simulink model "PLANET_v2"  (R2018b)
settings: Solver=FixedStepAuto  StartTime=0.0  StopTime=span-1  FixedStep=0.1  RelTol=1e-3
undefined symbols (not defined in the file): CHP_eta_el, CHP_eta_th, CHP_Pn, control, dh_demand, DH_elB_Cap, DH_elB_eff, DH_gas_B_Cap, DH_gas_B_eff, DH_HP_Cap, DH_HP_COP, DiscIntNeverNeededParam, dt, h_elD, lhd_demand, LHD_elB_Cap, LHD_elB_eff, LHD_gas_B_Cap, LHD_gas_B_eff, LHD_HP_Cap, LHD_HP_COP, Liion_cap, Liion_charge, Liion_dis, Liion_eff_ch, Liion_eff_dis, PCI, PtG_cap, PtG_eta_elcto, PtG_eta_meth, PtG_eta_th, PVPower, RES_curtailment_on_off, tt, WindPower
libraries: simulink x1
(part 1 of 5)
settings Model: Creator=Fambri  LastModifiedBy=gabriele.fambri
settings SolverCC: AlgebraicLoopSolver=LineSearch
settings DataIOCC: SaveFormat=StructureWithTime  SaveState=on  InspectSignalLogs=on
settings SFSimCC: SimUseLocalCustomCode=off
settings RTWCC: RTWUseLocalCustomCode=off
settings CodeAppCC: StateflowObjectComments=on

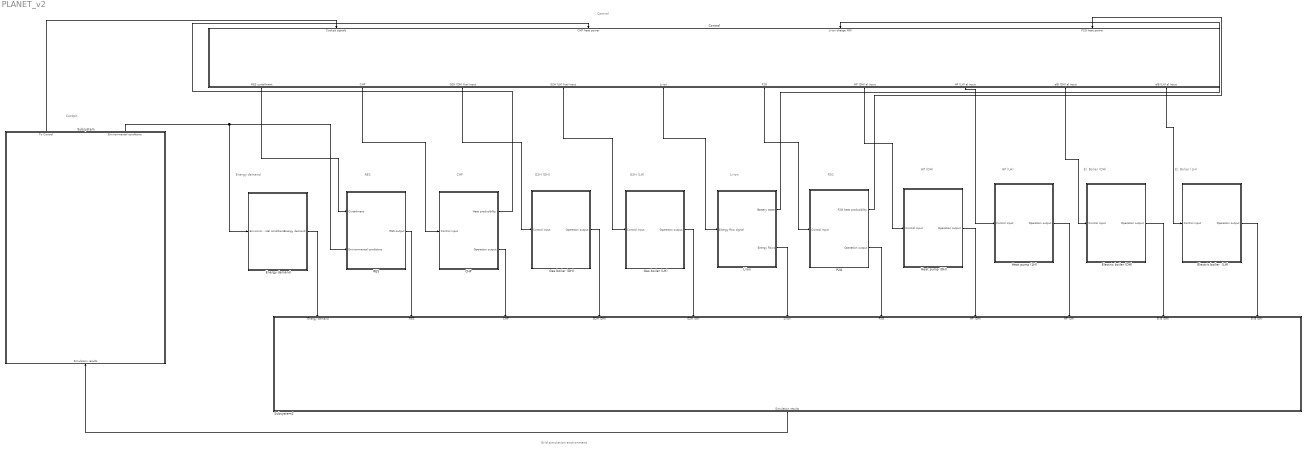
== system PLANET_v2 ==
  note: Li-ion
  note: Energy demand
  note: RES
  note: CHP
  note: P2G
  note: G2H (DH)
  note: Grid simulation environment
  note: Control
  note: HP (DH)
  note: Cockpit
  note: G2H (LH)
  note: HP (LH)
  note: El. Bolier (DH)
  note: El. Bolier (LH)
  CHP : Subsystem
  "Control " : Subsystem
  Electric boiler  (LH) : Subsystem
  Electric boiler (DH) : Subsystem
  Energy demand : Subsystem
  Gas boiler (DH) : Subsystem
  Gas boiler (LH) : Subsystem
  Heat pump (DH) : Subsystem
  Heat pump (LH) : Subsystem
  Liion : Subsystem
  P2G : Subsystem
  RES : Subsystem
  Subsystem : Subsystem
  Subsystem2 : Subsystem
  wires:
  Energy demand/1(Energy demand) -> Subsystem2/1(Energy demand)
  RES/1(RES output) -> Subsystem2/2(RES)
  Liion/2(Energy flows) -> Subsystem2/6(Li-ion)
  Gas boiler (DH)/1(Operation output) -> Subsystem2/4(G2H (DH))
  CHP/2(Operation output) -> Subsystem2/3(CHP)
  P2G/2(Operation output) -> Subsystem2/7(P2G)
  Subsystem/2(Environmental conditions) -> RES/2(Environmental conditions), Energy demand/1(Environmental conditions)
  Subsystem2/1(Simulation results) -> Subsystem/1(Simulation results)
  Subsystem/1(To Control) -> "Control "/1(Cockpit signals)
  P2G/1(P2G heat producibility) -> "Control "/4(P2G heat power)
  CHP/1(Heat producibility) -> "Control "/2(CHP heat power)
  Liion/1(Battery state) -> "Control "/3(Li-ion charge MW)
  "Control "/3("G2H (DH) fuel input ") -> Gas boiler (DH)/1(Control input)
  "Control "/1(RES curtailment) -> RES/1(Curtailment)
  "Control "/2(CHP) -> CHP/1(Control input)
  "Control "/6(P2G) -> P2G/1(Control input)
  "Control "/5(Li-ion) -> Liion/1(Energy flow signal)
  "Control "/7("HP (DH) el input ") -> Heat pump (DH)/1(Control input)
  Heat pump (DH)/1(Operation output) -> Subsystem2/8(HP (DH))
  "Control "/8("HP (LH) el input ") -> Heat pump (LH)/1(Control input)
  "Control "/9(elB (DH) el input) -> Electric boiler (DH)/1(Control input)
  "Control "/10(elB (LH) el input) -> Electric boiler  (LH)/1(Control input)
  "Control "/4(G2H (LH) fuel input) -> Gas boiler (LH)/1(Control input)
  Gas boiler (LH)/1(Operation output) -> Subsystem2/5(G2H (LH))
  Heat pump (LH)/1(Operation output) -> Subsystem2/9(HP (LH))
  Electric boiler (DH)/1(Operation output) -> Subsystem2/10(El B (DH))
  Electric boiler  (LH)/1(Operation output) -> Subsystem2/11(El B (LH))

== system PLANET_v2/CHP ==
  note: CHP fuel
  Control input : Inport
  Bus Creator : BusCreator  Inputs=3
  Bus Selector : BusSelector  OutputSignals=CHP fuel,CHP heat curtailment
  "CHP " : Subsystem  mask{PCI=PCI, eff_el=CHP_eta_el, Paus=0, eff_th=CHP_eta_th, Pn=CHP_Pn}
      mask prompts: PCI "PCI MWh/kg"; eff_el "Electric efficiency %"; Paus "Internal comsumption"; eff_th "Thermal efficiency %"; Pn "Nominal power MW"
  Sum : Sum  Inputs=|+-
  Heat producibility : Outport
  Operation output : Outport  Port=2
  wires:
  Bus Creator/1 -> Operation output/1
  "CHP "/3(Heat production) -> Heat producibility/1, Sum/1
  Sum/1 -> Bus Creator/3  "CHP heat power"
  Bus Selector/2 -> Sum/2  "<CHP heat curtailment>"
  "CHP "/1(Fuel consumption) -> Bus Creator/1
  Bus Selector/1 -> "CHP "/1(Fuel mass signal)  "<CHP fuel>"
  "CHP "/2(El production) -> Bus Creator/2  "CHP el power"
  Control input/1 -> Bus Selector/1

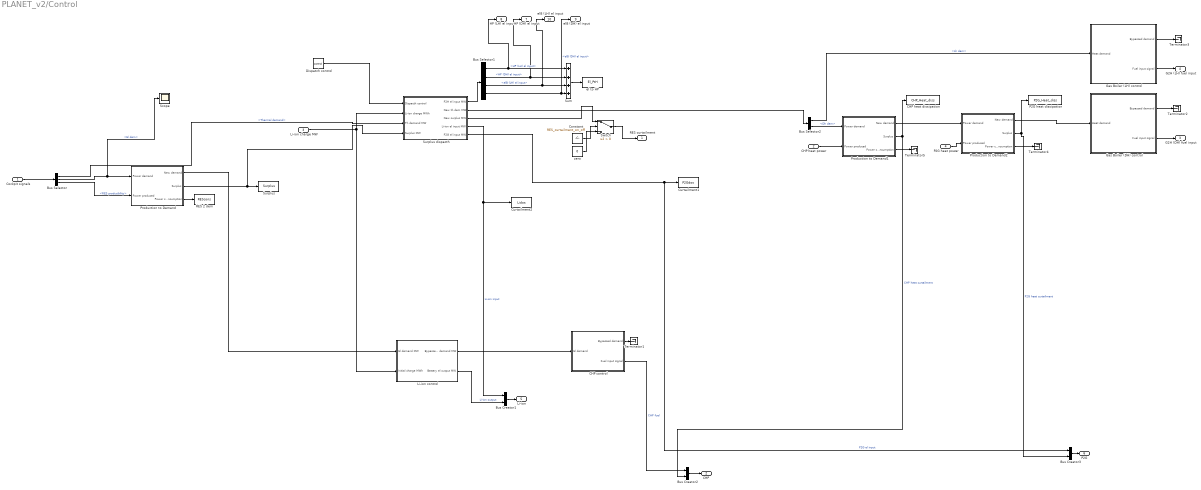
== system PLANET_v2/Control  ==
  Cockpit signals : Inport
  CHP heat power : Inport  Port=2
  Li-ion charge MW : Inport  Port=3
  P2G heat power : Inport  Port=4
  Bus Creator1 : BusCreator  Inputs=2
  Bus Creator2 : BusCreator  Inputs=2
  Bus Creator3 : BusCreator  Inputs=2
  Bus Selector : BusSelector  OutputSignals=Energy demand.Thermal demand,Energy demand.El dem,RES.RES producibility
  Bus Selector1 : BusSelector  OutputSignals=HP (LH) el input,HP (DH) el input,elB (LH) el input,elB (DH) el input
  Bus Selector2 : BusSelector  OutputSignals=Lh dem,Dh dem
  CHP control : Subsystem  mask{PCI=PCI, eff_el=CHP_eta_el, Paus=0, eff_th=CHP_eta_th, Pn=CHP_Pn}
      mask prompts: PCI "PCI MWh/kg"; eff_el "Electric efficiency %"; Paus "Internal comsumption"; eff_th "Thermal efficiency %"; Pn "Nominal power MW"
  CHP heat dissipation : ToWorkspace  VariableName=CHP_Heat_diss  SampleTime=1
  Constant : Constant  Value=RES_curtailment_on_off
  Curtailment1 : ToWorkspace  VariableName=P2Gdos  SampleTime=1
  Curtailment2 : ToWorkspace  VariableName=Lidos  SampleTime=1
  Dispatch control : Constant  Value=control
  Gas Boiler (DH) control : Subsystem  mask{PCI=PCI, eff=DH_gas_B_eff, Pn=DH_gas_B_Cap}
      mask prompts: PCI "PCI MWh/kg"; eff "Thermal efficiency %"; Pn "Nominal Power MW"
  Gas Boiler (LH) control : Subsystem  mask{PCI=PCI, eff=LHD_gas_B_eff, Pn=LHD_gas_B_Cap}
      mask prompts: PCI "PCI MWh/kg"; eff "Thermal efficiency %"; Pn "Nominal Power MW"
  Li-ion control : Subsystem  mask{eff_charge=Liion_eff_ch, eff_discharge=Liion_eff_dis, SoC_MAX=100, SoC_MIN=0, Capacity=Liion_cap, Initial_SoC=50, Max_charge=Liion_charge, Max_discharge=Liion_dis}
      mask prompts: eff_charge "charging efficiency [%]"; eff_discharge "discharging efficiency [%]"; SoC_MAX "Maximum state of charge [%]"; SoC_MIN "Minimum state of charge [%]"; Capacity "Capacity [MWh]"; Initial_SoC "Initial State of charge [%]"; Max_charge "Max charge [MW]"; Max_discharge "Max discharge [MW]"
  P2G heat dissipation : ToWorkspace  VariableName=P2G_Heat_diss  SampleTime=1
  Production to Demand : Subsystem
  Production to Demand1 : Subsystem
  Production to Demand2 : Subsystem
  RES 2 dem : ToWorkspace  VariableName=REScons  SampleTime=1
  Scope : Scope
  Sum : Sum  Inputs=++++
  Surplus : ToWorkspace  VariableName=Surplus  SampleTime=1
  Surplus dispacth : Subsystem
  Switch : Switch  Criteria=u2 > Threshold
  Terminator{1..5} (5 alike) : Terminator
  el to HP : ToWorkspace  VariableName=El_PtH  SampleTime=1
  zero : Constant  Value=0
  RES curtailment : Outport
  CHP : Outport  Port=2
  "G2H (DH) fuel input " : Outport  Port=3
  G2H (LH) fuel input : Outport  Port=4
  Li-ion : Outport  Port=5
  P2G : Outport  Port=6
  "HP (DH) el input " : Outport  Port=7
  "HP (LH) el input " : Outport  Port=8
  elB (DH) el input : Outport  Port=9
  elB (LH) el input : Outport  Port=10
  wires:
  Production to Demand/1(New demand) -> Li-ion control/1(El demand MW)
  Production to Demand/2(Surplus) -> Surplus dispacth/4(Surplus MW), Surplus/1
  Li-ion control/1(Bypassed demand MW) -> CHP control/1(El demand)
  Gas Boiler (DH) control/2(Fuel input signal) -> "G2H (DH) fuel input "/1
  Production to Demand1/2(Surplus) -> Bus Creator2/2, CHP heat dissipation/1  "CHP heat curtailment"
  Production to Demand2/1(New demand) -> Gas Boiler (DH) control/1(Heat demand)
  CHP control/2(Fuel input signal) -> Bus Creator2/1  "CHP fuel"
  Production to Demand2/2(Surplus) -> Bus Creator3/2, P2G heat dissipation/1  "P2G heat curtailment"
  P2G heat power/1 -> Production to Demand2/2(Power produced)
  Cockpit signals/1 -> Bus Selector/1
  Bus Creator2/1 -> CHP/1
  CHP heat power/1 -> Production to Demand1/2(Power produced)
  Bus Selector/3 -> Production to Demand/2(Power produced)  "<RES producibility>"
  Bus Creator1/1 -> Li-ion/1
  Li-ion control/2(Battery el output MW) -> Bus Creator1/2  "Li-ion output"
  Surplus dispacth/3(New surplus MW) -> Switch/1
  Li-ion charge MW/1 -> Li-ion control/2(Initial charge MWh), Surplus dispacth/2(Li-ion charge MWh)
  Surplus dispacth/1(P2H el input MW) -> Bus Selector1/1
  Surplus dispacth/4(Li-ion el input MW) -> Bus Creator1/1, Curtailment2/1  "Li-ion input"
  Surplus dispacth/5(P2G el input MW) -> Bus Creator3/1, Curtailment1/1  "P2G el input"
  Dispatch control/1 -> Surplus dispacth/1(Dispacth control)
  Production to Demand/3(Power consumption) -> RES 2 dem/1
  Bus Creator3/1 -> P2G/1
  Production to Demand1/1(New demand) -> Production to Demand2/1(Power demand)
  Bus Selector/2 -> Scope/1, Production to Demand/1(Power demand)  "<El dem>"
  Bus Selector/1 -> Surplus dispacth/3(Th demand MW)  "<Thermal demand>"
  Bus Selector1/2 -> Sum/2, "HP (DH) el input "/1  "<HP (DH) el input>"
  Bus Selector1/3 -> Sum/3, elB (LH) el input/1  "<elB (LH) el input>"
  Bus Selector1/4 -> elB (DH) el input/1, Sum/4  "<elB (DH) el input>"
  Sum/1 -> el to HP/1
  Surplus dispacth/2(New th dem MW) -> Bus Selector2/1
  Bus Selector2/2 -> Production to Demand1/1(Power demand)  "<Dh dem>"
  Bus Selector2/1 -> Gas Boiler (LH) control/1(Heat demand)  "<Lh dem>"
  Gas Boiler (LH) control/2(Fuel input signal) -> G2H (LH) fuel input/1
  Bus Selector1/1 -> "HP (LH) el input "/1, Sum/1  "<HP (LH) el input>"
  CHP control/1(Bypassed demand) -> Terminator1/1
  Gas Boiler (DH) control/1(Bypassed demand) -> Terminator2/1
  Gas Boiler (LH) control/1(Bypassed demand) -> Terminator3/1
  Production to Demand2/3(Power consumption) -> Terminator4/1
  Production to Demand1/3(Power consumption) -> Terminator5/1
  Constant/1 -> Switch/2
  zero/1 -> Switch/3
  Switch/1 -> RES curtailment/1

== system PLANET_v2/Electric boiler  (LH) ==
  Control input : Inport
  Bus Creator : BusCreator  Inputs=2
  Heat production : ToWorkspace  VariableName=h_P2H_elB_LH  SampleTime=1
  P2H : Subsystem  mask{COP=LHD_elB_eff, Cap=LHD_elB_Cap}
      mask prompts: COP "Efficiency/COP"; Cap "Capacity"
  Operation output : Outport
  wires:
  Control input/1 -> P2H/1(El input)
  P2H/2(heat) -> Bus Creator/2, Heat production/1  "elB (LH) heat production"
  P2H/1(El consumption) -> Bus Creator/1  "elB (LH) el input"
  Bus Creator/1 -> Operation output/1  "elB (LH) data"

== system PLANET_v2/Electric boiler (DH) ==
  Control input : Inport
  Bus Creator : BusCreator  Inputs=2
  Heat production : ToWorkspace  VariableName=h_P2H_elB_DH  SampleTime=1
  P2H : Subsystem  mask{COP=DH_elB_eff, Cap=DH_elB_Cap}
      mask prompts: COP "Efficiency/COP"; Cap "Capacity"
  Operation output : Outport
  wires:
  Control input/1 -> P2H/1(El input)
  P2H/2(heat) -> Heat production/1, Bus Creator/2  "elB (DH) heat production"
  P2H/1(El consumption) -> Bus Creator/1  "elB (DH) el input"
  Bus Creator/1 -> Operation output/1  "elB (DH) data"

== system PLANET_v2/Energy demand ==
  Environmental conditions : Inport
  Bus Creator : BusCreator  Inputs=2
  Bus Creator1 : BusCreator  Inputs=2
  Bus Selector : BusSelector  OutputSignals=El dem,DH standar profile,LH standard profile
  DH demand : Subsystem
  El demand : Subsystem
  LH demand : Subsystem
  Energy demand : Outport
  wires:
  Environmental conditions/1 -> Bus Selector/1
  DH demand/1(DH demand) -> Bus Creator1/1  "Dh dem"
  Bus Creator/1 -> Energy demand/1
  Bus Selector/1 -> El demand/1(In1)  "<El dem>"
  El demand/1(El demand) -> Bus Creator/1  "El dem"
  LH demand/1(DH demand) -> Bus Creator1/2  "Lh dem"
  Bus Creator1/1 -> Bus Creator/2  "Thermal demand"
  Bus Selector/2 -> DH demand/1(In1)  "<DH standar profile>"
  Bus Selector/3 -> LH demand/1(In1)  "<LH standard profile>"

== system PLANET_v2/Gas boiler (DH) ==
  Control input : Inport
  Bus Creator : BusCreator  Inputs=2
  DH Gas Boiler block : Subsystem  mask{PCI=PCI, eff=DH_gas_B_eff, Pn=DH_gas_B_Cap}
      mask prompts: PCI "PCI MWh/kg"; eff "Thermal efficiency %"; Pn "Nominal Power MW"
  Operation output : Outport
  wires:
  Bus Creator/1 -> Operation output/1  "G2H (DH) data"
  DH Gas Boiler block/2(Thermal power) -> Bus Creator/2  "DG2H heat"
  DH Gas Boiler block/1("Fuel mass ") -> Bus Creator/1  "DG2H fuel"
  Control input/1 -> DH Gas Boiler block/1(Fuel mass signal)

== system PLANET_v2/Gas boiler (LH) ==
  Control input : Inport
  Bus Creator : BusCreator  Inputs=2
  LH Gas Boiler block : Subsystem  mask{PCI=PCI, eff=LHD_gas_B_eff, Pn=LHD_gas_B_Cap}
      mask prompts: PCI "PCI MWh/kg"; eff "Thermal efficiency %"; Pn "Nominal Power MW"
  Operation output : Outport
  wires:
  Bus Creator/1 -> Operation output/1  "G2H (LH) data"
  LH Gas Boiler block/2(Thermal power) -> Bus Creator/2  "LG2H heat"
  LH Gas Boiler block/1("Fuel mass ") -> Bus Creator/1  "LG2H fuel"
  Control input/1 -> LH Gas Boiler block/1(Fuel mass signal)

== system PLANET_v2/Heat pump (DH) ==
  Control input : Inport
  Bus Creator : BusCreator  Inputs=2
  Heat production : ToWorkspace  VariableName=h_P2H_HP_DH  SampleTime=1
  P2H : Subsystem  mask{COP=DH_HP_COP, Cap=DH_HP_Cap}
      mask prompts: COP "Efficiency/COP"; Cap "Capacity"
  Operation output : Outport
  wires:
  Control input/1 -> P2H/1(El input)
  P2H/2(heat) -> Heat production/1, Bus Creator/2  "DHP heat production"
  P2H/1(El consumption) -> Bus Creator/1  "DHP el input"
  Bus Creator/1 -> Operation output/1  "HP (DH) data"

== system PLANET_v2/Heat pump (LH) ==
  Control input : Inport
  Bus Creator : BusCreator  Inputs=2
  Heat production : ToWorkspace  VariableName=h_P2H_HP_LH  SampleTime=1
  P2H : Subsystem  mask{COP=LHD_HP_COP, Cap=LHD_HP_Cap}
      mask prompts: COP "Efficiency/COP"; Cap "Capacity"
  Operation output : Outport
  wires:
  Control input/1 -> P2H/1(El input)
  P2H/2(heat) -> Heat production/1, Bus Creator/2  "LHP heat production"
  P2H/1(El consumption) -> Bus Creator/1  "LHP el input"
  Bus Creator/1 -> Operation output/1  "HP (LH) data"

== system PLANET_v2/Liion ==
  note: Li-ion input
  Energy flow signal : Inport
  Bus Creator : BusCreator  Inputs=2
  Bus Selector : BusSelector  OutputSignals=Li-ion input,Li-ion output
  "Li-ion " : Subsystem  mask{eff_charge=Liion_eff_ch, eff_discharge=Liion_eff_dis, SoC_MAX=100, SoC_MIN=0, Capacity=Liion_cap, Initial_SoC=50, Max_charge=Liion_charge, Max_discharge=Liion_dis, Parameter11=<empty>}
      mask prompts: eff_charge "charging efficiency [%]"; eff_discharge "discharging efficiency [%]"; SoC_MAX "Maximum state of charge [%]"; SoC_MIN "Minimum state of charge [%]"; Capacity "Capacity [MWh]"; Initial_SoC "Initial State of charge [%]"; Max_charge "Max charge [MW]"; Max_discharge "Max discharge [MW]"
      mask TypeOptions Parameter11: <empty>
  Battery state : Outport
  Energy flows : Outport  Port=2
  wires:
  Energy flow signal/1 -> Bus Selector/1
  "Li-ion "/1(Initial Charge) -> Battery state/1
  Bus Creator/1 -> Energy flows/1
  "Li-ion "/2(El consumption) -> Bus Creator/1
  "Li-ion "/3(El production) -> Bus Creator/2  "Li-ion output"
  Bus Selector/1 -> "Li-ion "/1(El input)  "<Li-ion input>"
  Bus Selector/2 -> "Li-ion "/2(El output)  "<Li-ion output>"

== system PLANET_v2/P2G ==
  Control input : Inport
  Bus Creator : BusCreator  Inputs=3
  Bus Selector : BusSelector  OutputSignals=P2G el input,P2G heat curtailment
  P2G : Subsystem  mask{PtG_capacity=PtG_cap, eff_electrolyser=PtG_eta_elcto, eff_methanizer=PtG_eta_meth, eff_thermal=PtG_eta_th, PCI=PCI}
      mask prompts: PtG_capacity "PtG capacity"; eff_electrolyser "Electrolyser efficiency"; eff_methanizer "Methanizer efficiency"; eff_thermal "Thermal efficiency"; PCI "PCI Mehtane MWh/kg"
  Sum2 : Sum  Inputs=|+-
  P2G heat producibility : Outport
  Operation output : Outport  Port=2
  wires:
  Bus Creator/1 -> Operation output/1
  P2G/2(El consumption) -> Bus Creator/2  "P2G el imput"
  Sum2/1 -> Bus Creator/3  "P2G heat production"
  Bus Selector/2 -> Sum2/2  "<P2G heat curtailment>"
  P2G/1(Gas productioon) -> Bus Creator/1  "P2G gas production"
  P2G/3(Heat production) -> P2G heat producibility/1, Sum2/1
  Bus Selector/1 -> P2G/1(El input)  "<P2G el input>"
  Control input/1 -> Bus Selector/1

== system PLANET_v2/RES ==
  Curtailment : Inport
  Environmental conditions : Inport  Port=2
  Bus Creator : BusCreator  Inputs=3
  Bus Selector : BusSelector  OutputSignals=Wind,PV,Hydro
  Subsystem : Subsystem
  Sum1 : Sum  Inputs=-+|
  Sum3 : Sum  Inputs=+++
  RES output : Outport
  wires:
  Sum3/1 -> Sum1/2, Bus Creator/3  "RES producibility"
  Subsystem/2(RES2) -> Sum3/2
  Subsystem/1(RES1) -> Sum3/1
  Subsystem/3(RES3) -> Sum3/3
  Bus Selector/1 -> Subsystem/1(Wind)  "<Wind>"
  Bus Selector/2 -> Subsystem/2(PV)  "<PV>"
  Sum1/1 -> Bus Creator/2  "RES production"
  Curtailment/1 -> Bus Creator/1, Sum1/1  "Curtailment"
  Bus Creator/1 -> RES output/1
  Environmental conditions/1 -> Bus Selector/1
  Bus Selector/3 -> Subsystem/3(Hydro)  "<Hydro>"

== system PLANET_v2/Subsystem ==
  Simulation results : Inport
  Environment : Subsystem
  To Matlab : Subsystem
  To Control : Outport
  Environmental conditions : Outport  Port=2
  wires:
  Simulation results/1 -> To Matlab/1(Simulation results), To Control/1
  Environment/1(Environmental conditions) -> Environmental conditions/1

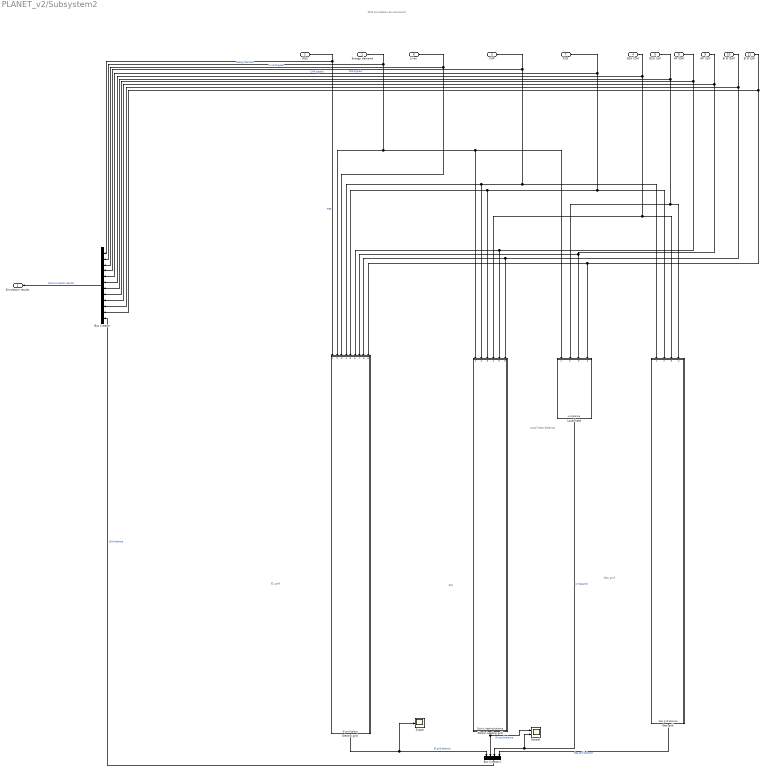
== system PLANET_v2/Subsystem2 ==
  note: EL grid
  note: DH
  note: Local heat balance
  note: Gas grid
  note: Grid simulation environment
  Energy demand : Inport
  RES : Inport  Port=2
  CHP : Inport  Port=3
  G2H (DH) : Inport  Port=4
  G2H (LH) : Inport  Port=5
  Li-ion : Inport  Port=6
  P2G : Inport  Port=7
  HP (DH) : Inport  Port=8
  HP (LH) : Inport  Port=9
  El B (DH) : Inport  Port=10
  El B (LH) : Inport  Port=11
  Bus Creator : BusCreator  Inputs=12
  Bus Creator1 : BusCreator  Inputs=4
  Distric heating grid : Subsystem
  Electric grid : Subsystem
  Gas grid : Subsystem
  Local heat : Subsystem
  Scope : Scope
  Scope1 : Scope  NumInputPorts=2
  Simulation results : Outport
  wires:
  G2H (DH)/1 -> Gas grid/3(Gas boiler (DH)), Distric heating grid/4(Gas boiler (DH)), Bus Creator/6
  Bus Creator/1 -> Simulation results/1  "Grid simulation results"
  Electric grid/1(El grid balace) -> Scope/1, Bus Creator1/1  "El grid balance"
  Energy demand/1 -> Distric heating grid/1(Demand consumption), Local heat/1(LH dem), Electric grid/2(Demand consumption), Bus Creator/2  "Energy demand"
  CHP/1 -> Gas grid/1(CHP consumption), Electric grid/4(CHP production), Distric heating grid/2(CHP production), Bus Creator/4  "CHP signals"
  Bus Creator1/1 -> Bus Creator/12  "Grid balance"
  P2G/1 -> Electric grid/5(P2G consumption), Distric heating grid/3(P2G production), Gas grid/2(P2G production), Bus Creator/5  "P2G signals"
  Distric heating grid/1(Distric heating balance) -> Scope1/1, Bus Creator1/2  "DH grid balance"
  Gas grid/1(Gas grid balance) -> Bus Creator1/4  "Gas grid balance"
  Li-ion/1 -> Electric grid/3(Li-ion), Bus Creator/3  "Li-ion signals"
  HP (DH)/1 -> Electric grid/6(HP (DH) el), Distric heating grid/5(HP (DH)), Bus Creator/8
  RES/1 -> Bus Creator/1, Electric grid/1(RES)  "RES"
  Local heat/1(LH balance) -> Scope1/2, Bus Creator1/3  "LH balance"
  G2H (LH)/1 -> Local heat/2(Gas boiler (LH)), Gas grid/4(Gas boiler (LH)), Bus Creator/7
  HP (LH)/1 -> Local heat/3(HP (LH)), Electric grid/7(HP (LH) el), Bus Creator/9
  El B (DH)/1 -> Electric grid/8(El B (DH) el), Distric heating grid/6(El B (DH)), Bus Creator/10
  El B (LH)/1 -> Electric grid/9(El B (LH) el), Local heat/4(El B (LH)), Bus Creator/11

== system PLANET_v2/CHP/CHP  ==
  Fuel mass signal : Inport
  CHP : Subsystem
  Fuel consumption : Outport
  El production : Outport  Port=2
  Heat production : Outport  Port=3
  wires:
  CHP/1(Electric power) -> El production/1
  Fuel mass signal/1 -> Fuel consumption/1, CHP/1(Fuel mass flow rate)
  CHP/2(Thermal power) -> Heat production/1

== system PLANET_v2/Control /CHP control ==
  El demand : Inport
  Divide1 : Product  Inputs=*/
  Divide2 : Product  Inputs=**
  Electric efficiency : Constant  Value=eff_el/100
  Internal comsumption : Constant  Value=Paus
  Nominal CHP power : Constant  Value=Pn
  PCI MJ/kg1 : Constant  Value=PCI
  Saturation : Saturate  UpperLimit=Pn/PCI/(eff_el/100)  LowerLimit=0
  Saturation1 : Saturate  UpperLimit=inf  LowerLimit=0
  Sum1 : Sum  Inputs=++|
  Sum2 : Sum  Inputs=-+|
  Bypassed demand : Outport
  Fuel input signal : Outport  Port=2
  wires:
  Sum1/1 -> Divide1/1
  Internal comsumption/1 -> Sum1/1
  Electric efficiency/1 -> Divide2/2
  Sum2/1 -> Saturation1/1
  Saturation/1 -> Fuel input signal/1
  El demand/1 -> Sum2/2, Sum1/2
  Saturation1/1 -> Bypassed demand/1
  PCI MJ/kg1/1 -> Divide2/1
  Divide2/1 -> Divide1/2
  Nominal CHP power/1 -> Sum2/1
  Divide1/1 -> Saturation/1

== system PLANET_v2/Control /Gas Boiler (DH) control ==
  Heat demand : Inport
  Divide1 : Product  Inputs=*/
  Divide2 : Product  Inputs=**
  Nominal Gas boiler power : Constant  Value=Pn
  PCI MJ/kg1 : Constant  Value=PCI
  Saturation : Saturate  UpperLimit=Pn/PCI/(eff/100)  LowerLimit=0
  Saturation1 : Saturate  UpperLimit=inf  LowerLimit=0
  Sum4 : Sum  Inputs=-+|
  thermal efficiency : Constant  Value=eff/100
  Bypassed demand : Outport
  Fuel input signal : Outport  Port=2
  wires:
  Divide1/1 -> Saturation/1
  Divide2/1 -> Divide1/2
  Saturation/1 -> Fuel input signal/1
  Sum4/1 -> Saturation1/1
  PCI MJ/kg1/1 -> Divide2/1
  Saturation1/1 -> Bypassed demand/1
  thermal efficiency/1 -> Divide2/2
  Nominal Gas boiler power/1 -> Sum4/1
  Heat demand/1 -> Divide1/1, Sum4/2

== system PLANET_v2/Control /Gas Boiler (LH) control ==
  Heat demand : Inport
  Divide1 : Product  Inputs=*/
  Divide2 : Product  Inputs=**
  Nominal Gas boiler power : Constant  Value=Pn
  PCI MJ/kg1 : Constant  Value=PCI
  Saturation : Saturate  UpperLimit=Pn/PCI/(eff/100)  LowerLimit=0
  Saturation1 : Saturate  UpperLimit=inf  LowerLimit=0
  Scope : Scope  NumInputPorts=2
  Sum4 : Sum  Inputs=-+|
  thermal efficiency : Constant  Value=eff/100
  Bypassed demand : Outport
  Fuel input signal : Outport  Port=2
  wires:
  Divide1/1 -> Scope/1, Saturation/1
  Divide2/1 -> Divide1/2
  Saturation/1 -> Scope/2, Fuel input signal/1
  Sum4/1 -> Saturation1/1
  PCI MJ/kg1/1 -> Divide2/1
  Saturation1/1 -> Bypassed demand/1
  thermal efficiency/1 -> Divide2/2
  Nominal Gas boiler power/1 -> Sum4/1
  Heat demand/1 -> Divide1/1, Sum4/2

== system PLANET_v2/Control /Li-ion control ==
  El demand MW : Inport
  Initial charge MWh : Inport  Port=2
  Available Energy MWh : Subsystem
  Bypassed dem : Merge  Inputs=4
  Disch eff : Gain  Gain=eff_discharge/100
  Energy to Power : Subsystem
  From battery : Merge  Inputs=4
  If Action Subsystem3 : Subsystem  TreatAsAtomicUnit=on
  If Action Subsystem5 : Subsystem  TreatAsAtomicUnit=on
  If Action Subsystem6 : Subsystem  TreatAsAtomicUnit=on
  If Action Subsystem7 : Subsystem  TreatAsAtomicUnit=on
  Max discharge rate MW : Subsystem
  if demand : If  NumInputs=3  IfExpression=u1 == 0  ElseIfExpressions=(u1 <= u2) & (u1<=u3), u2<=u3
  Bypassed demand MW : Outport
  Battery el output MW : Outport  Port=2
  wires:
  if demand/4 -> If Action Subsystem7/Action
  Bypassed dem/1 -> Bypassed demand MW/1  "Unsatisfied demandt"
  If Action Subsystem5/1(From battery) -> From battery/2
  Available Energy MWh/1(Charge available) -> Energy to Power/1(Energy)
  if demand/1 -> If Action Subsystem3/Action
  If Action Subsystem7/2(Bypassed demand) -> Bypassed dem/4
  Max discharge rate MW/1(Max battery discharge) -> If Action Subsystem6/1(Max discharge), if demand/2
  If Action Subsystem5/2(Bypassed demand) -> Bypassed dem/2
  if demand/2 -> If Action Subsystem5/Action
  From battery/1 -> Battery el output MW/1  "Energy coming from the battery"
  If Action Subsystem6/2(Bypassed demand) -> Bypassed dem/3
  If Action Subsystem7/1(From battery) -> From battery/4
  if demand/3 -> If Action Subsystem6/Action
  If Action Subsystem3/2("Bypassed demand ") -> Bypassed dem/1
  If Action Subsystem6/1(From battery) -> From battery/3
  If Action Subsystem3/1(From battery) -> From battery/1
  El demand MW/1 -> If Action Subsystem7/2(Demnad), If Action Subsystem6/2(Demand), if demand/1, If Action Subsystem5/1(Demand)
  Initial charge MWh/1 -> Available Energy MWh/1(In1)
  Energy to Power/1(Power) -> Disch eff/1
  Disch eff/1 -> If Action Subsystem7/1(Available battery), if demand/3

== system PLANET_v2/Control /Production to Demand ==
  Power demand : Inport
  Power produced : Inport  Port=2
  If : If  NumInputs=2  IfExpression=u1 >= u2
  If Action Subsystem : Subsystem  TreatAsAtomicUnit=on
  If Action Subsystem1 : Subsystem  TreatAsAtomicUnit=on
  Merge : Merge
  Merge1 : Merge
  Sum : Sum  Inputs=|+-
  New demand : Outport
  Surplus : Outport  Port=2
  Power consumption : Outport  Port=3
  wires:
  Power demand/1 -> If Action Subsystem1/2(Power demand), If Action Subsystem/2(Power demand), If/2
  Power produced/1 -> Sum/1, If Action Subsystem1/1(Power produced), If Action Subsystem/1(Power produced), If/1
  If/1 -> If Action Subsystem/Action
  If/2 -> If Action Subsystem1/Action
  Merge/1 -> Sum/2, Surplus/1
  If Action Subsystem/2(Surplus) -> Merge/1
  If Action Subsystem1/1(Surplus) -> Merge/2
  If Action Subsystem/1(New demand) -> Merge1/1
  If Action Subsystem1/2(New demand) -> Merge1/2
  Merge1/1 -> New demand/1
  Sum/1 -> Power consumption/1

== system PLANET_v2/Control /Production to Demand1 ==
  Power demand : Inport
  Power produced : Inport  Port=2
  If : If  NumInputs=2  IfExpression=u1 >= u2
  If Action Subsystem : Subsystem  TreatAsAtomicUnit=on
  If Action Subsystem1 : Subsystem  TreatAsAtomicUnit=on
  Merge : Merge
  Merge1 : Merge
  Sum : Sum  Inputs=|+-
  New demand : Outport
  Surplus : Outport  Port=2
  Power consumption : Outport  Port=3
  wires:
  Power demand/1 -> If Action Subsystem1/2(Power demand), If Action Subsystem/2(Power demand), If/2
  Power produced/1 -> Sum/1, If Action Subsystem1/1(Power produced), If Action Subsystem/1(Power produced), If/1
  If/1 -> If Action Subsystem/Action
  If/2 -> If Action Subsystem1/Action
  Merge/1 -> Sum/2, Surplus/1
  If Action Subsystem/2(Surplus) -> Merge/1
  If Action Subsystem1/1(Surplus) -> Merge/2
  If Action Subsystem/1(New demand) -> Merge1/1
  If Action Subsystem1/2(New demand) -> Merge1/2
  Merge1/1 -> New demand/1
  Sum/1 -> Power consumption/1

== system PLANET_v2/Control /Production to Demand2 ==
  Power demand : Inport
  Power produced : Inport  Port=2
  If : If  NumInputs=2  IfExpression=u1 >= u2
  If Action Subsystem : Subsystem  TreatAsAtomicUnit=on
  If Action Subsystem1 : Subsystem  TreatAsAtomicUnit=on
  Merge : Merge
  Merge1 : Merge
  Sum : Sum  Inputs=|+-
  New demand : Outport
  Surplus : Outport  Port=2
  Power consumption : Outport  Port=3
  wires:
  Power demand/1 -> If Action Subsystem1/2(Power demand), If Action Subsystem/2(Power demand), If/2
  Power produced/1 -> Sum/1, If Action Subsystem1/1(Power produced), If Action Subsystem/1(Power produced), If/1
  If/1 -> If Action Subsystem/Action
  If/2 -> If Action Subsystem1/Action
  Merge/1 -> Sum/2, Surplus/1
  If Action Subsystem/2(Surplus) -> Merge/1
  If Action Subsystem1/1(Surplus) -> Merge/2
  If Action Subsystem/1(New demand) -> Merge1/1
  If Action Subsystem1/2(New demand) -> Merge1/2
  Merge1/1 -> New demand/1
  Sum/1 -> Power consumption/1

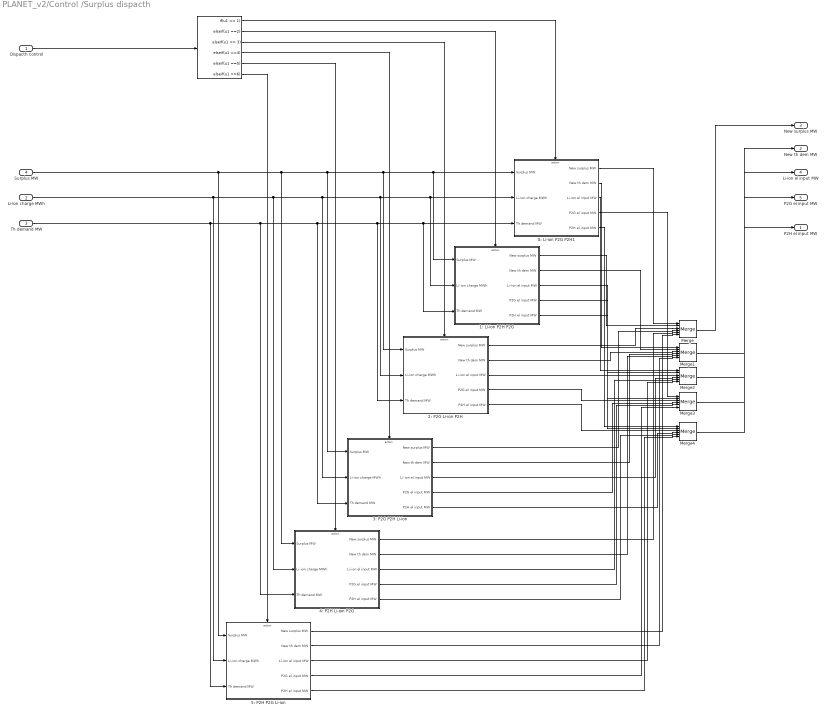
== system PLANET_v2/Control /Surplus dispacth ==
  Dispacth control : Inport
  Li-ion charge MWh : Inport  Port=2
  Th demand MW : Inport  Port=3
  Surplus MW : Inport  Port=4
  " " : If  IfExpression=u1 == 1  ElseIfExpressions=u1 ==2, u1 == 3, u1 ==4, u1 ==5, u1 ==6  ShowElse=off
  0: Li-ion P2G P2H1 : Subsystem  TreatAsAtomicUnit=on
  1: Li-ion P2H P2G : Subsystem  TreatAsAtomicUnit=on
  2: P2G Li-ion P2H : Subsystem  TreatAsAtomicUnit=on
  3: P2G P2H Li-ion : Subsystem  TreatAsAtomicUnit=on
  4: P2H Li-ion P2G : Subsystem  TreatAsAtomicUnit=on
  "5: P2H P2G Li-ion " : Subsystem  TreatAsAtomicUnit=on
  Merge{,1..4} (5 alike) : Merge  Inputs=6
  P2H el input MW : Outport
  New th dem MW : Outport  Port=2
  New surplus MW : Outport  Port=3
  Li-ion el input MW : Outport  Port=4
  P2G el input MW : Outport  Port=5
  wires:
  Merge/1 -> New surplus MW/1
  Dispacth control/1 -> " "/1
  " "/6 -> "5: P2H P2G Li-ion "/Action
  " "/5 -> 4: P2H Li-ion P2G/Action
  " "/4 -> 3: P2G P2H Li-ion/Action
  " "/3 -> 2: P2G Li-ion P2H/Action
  " "/2 -> 1: Li-ion P2H P2G/Action
  " "/1 -> 0: Li-ion P2G P2H1/Action
  Merge4/1 -> P2H el input MW/1
  Merge3/1 -> P2G el input MW/1
  Merge2/1 -> Li-ion el input MW/1
  Merge1/1 -> New th dem MW/1
  "5: P2H P2G Li-ion "/5(P2H el input MW) -> Merge4/6
  1: Li-ion P2H P2G/5(P2H el input MW) -> Merge4/2
  4: P2H Li-ion P2G/5(P2H el input MW) -> Merge4/5
  3: P2G P2H Li-ion/5(P2H el input MW) -> Merge4/4
  2: P2G Li-ion P2H/5(P2H el input MW) -> Merge4/3
  0: Li-ion P2G P2H1/5(P2H el input MW) -> Merge4/1
  "5: P2H P2G Li-ion "/4(P2G el input MW) -> Merge3/6
  4: P2H Li-ion P2G/4(P2G el input MW) -> Merge3/5
  3: P2G P2H Li-ion/4(P2G el input MW) -> Merge3/4
  2: P2G Li-ion P2H/4(P2G el input MW) -> Merge3/3
  1: Li-ion P2H P2G/4(P2G el input MW) -> Merge3/2
  0: Li-ion P2G P2H1/4(P2G el input MW) -> Merge3/1
  "5: P2H P2G Li-ion "/3(Li-ion el input MW) -> Merge2/6
  4: P2H Li-ion P2G/3(Li-ion el input MW) -> Merge2/5
  3: P2G P2H Li-ion/3(Li-ion el input MW) -> Merge2/4
  2: P2G Li-ion P2H/3(Li-ion el input MW) -> Merge2/3
  1: Li-ion P2H P2G/3(Li-ion el input MW) -> Merge2/2
  0: Li-ion P2G P2H1/3(Li-ion el input MW) -> Merge2/1
  "5: P2H P2G Li-ion "/2(New th dem MW) -> Merge1/6
  4: P2H Li-ion P2G/2(New th dem MW) -> Merge1/5
  3: P2G P2H Li-ion/2(New th dem MW) -> Merge1/4
  2: P2G Li-ion P2H/2(New th dem MW) -> Merge1/3
  1: Li-ion P2H P2G/2(New th dem MW) -> Merge1/2
  0: Li-ion P2G P2H1/2(New th dem MW) -> Merge1/1
  "5: P2H P2G Li-ion "/1(New surplus MW) -> Merge/6
  4: P2H Li-ion P2G/1(New surplus MW) -> Merge/5
  3: P2G P2H Li-ion/1(New surplus MW) -> Merge/4
  2: P2G Li-ion P2H/1(New surplus MW) -> Merge/3
  1: Li-ion P2H P2G/1(New surplus MW) -> Merge/2
  0: Li-ion P2G P2H1/1(New surplus MW) -> Merge/1
  Th demand MW/1 -> 0: Li-ion P2G P2H1/3(Th demand MW), 1: Li-ion P2H P2G/3(Th demand MW), 2: P2G Li-ion P2H/3(Th demand MW), 3: P2G P2H Li-ion/3(Th demand MW), 4: P2H Li-ion P2G/3(Th demand MW), "5: P2H P2G Li-ion "/3(Th demand MW)
  Li-ion charge MWh/1 -> 0: Li-ion P2G P2H1/2(" Li-ion charge MWh"), 1: Li-ion P2H P2G/2(" Li-ion charge MWh"), 2: P2G Li-ion P2H/2(" Li-ion charge MWh"), 3: P2G P2H Li-ion/2(" Li-ion charge MWh"), 4: P2H Li-ion P2G/2(" Li-ion charge MWh"), "5: P2H P2G Li-ion "/2(" Li-ion charge MWh")
  Surplus MW/1 -> 0: Li-ion P2G P2H1/1(Surplus MW), 1: Li-ion P2H P2G/1(Surplus MW), 2: P2G Li-ion P2H/1(Surplus MW), 3: P2G P2H Li-ion/1(Surplus MW), 4: P2H Li-ion P2G/1(Surplus MW), "5: P2H P2G Li-ion "/1(Surplus MW)

== system PLANET_v2/Electric boiler  (LH)/P2H ==
  El input : Inport
  Gain : Gain  Gain=COP
  Saturation : Saturate  UpperLimit=Cap  LowerLimit=0
  El consumption : Outport
  heat : Outport  Port=2
  wires:
  Gain/1 -> heat/1
  Saturation/1 -> Gain/1
  El input/1 -> El consumption/1, Saturation/1

== system PLANET_v2/Electric boiler (DH)/P2H ==
  El input : Inport
  Gain : Gain  Gain=COP
  Saturation : Saturate  UpperLimit=Cap  LowerLimit=0
  El consumption : Outport
  heat : Outport  Port=2
  wires:
  Gain/1 -> heat/1
  Saturation/1 -> Gain/1
  El input/1 -> El consumption/1, Saturation/1

== system PLANET_v2/Energy demand/DH demand ==
  In1 : Inport
  DH demand : Outport
  wires:
  In1/1 -> DH demand/1

== system PLANET_v2/Energy demand/El demand ==
  In1 : Inport
  El demand : Outport
  wires:
  In1/1 -> El demand/1

== system PLANET_v2/Energy demand/LH demand ==
  In1 : Inport
  DH demand : Outport
  wires:
  In1/1 -> DH demand/1

== system PLANET_v2/Gas boiler (DH)/DH Gas Boiler block ==
  Fuel mass signal : Inport
  Boiler : Subsystem
  Saturation : Saturate  UpperLimit=Pn/PCI/(eff/100)  LowerLimit=0
  "Fuel mass " : Outport
  Thermal power : Outport  Port=2
  wires:
  Boiler/1(Thermal power) -> Thermal power/1
  Fuel mass signal/1 -> Saturation/1
  Saturation/1 -> "Fuel mass "/1, Boiler/1(Fuel mass)

== system PLANET_v2/Gas boiler (LH)/LH Gas Boiler block ==
  Fuel mass signal : Inport
  Boiler : Subsystem
  Saturation : Saturate  UpperLimit=Pn/PCI/(eff/100)  LowerLimit=0
  "Fuel mass " : Outport
  Thermal power : Outport  Port=2
  wires:
  Boiler/1(Thermal power) -> Thermal power/1
  Saturation/1 -> "Fuel mass "/1, Boiler/1(Fuel mass)
  Fuel mass signal/1 -> Saturation/1

== system PLANET_v2/Heat pump (DH)/P2H ==
  El input : Inport
  Gain : Gain  Gain=COP
  Saturation : Saturate  UpperLimit=Cap  LowerLimit=0
  El consumption : Outport
  heat : Outport  Port=2
  wires:
  Gain/1 -> heat/1
  Saturation/1 -> Gain/1
  El input/1 -> El consumption/1, Saturation/1

== system PLANET_v2/Heat pump (LH)/P2H ==
  El input : Inport
  Gain : Gain  Gain=COP
  Saturation : Saturate  UpperLimit=Cap  LowerLimit=0
  El consumption : Outport
  heat : Outport  Port=2
  wires:
  Gain/1 -> heat/1
  Saturation/1 -> Gain/1
  El input/1 -> El consumption/1, Saturation/1

== system PLANET_v2/Liion/Li-ion  ==
  El input : Inport
  El output : Inport  Port=2
  1/Dis eff : Gain  Gain=100/eff_discharge
  Ch eff : Gain  Gain=eff_charge/100
  Li-ion Charge : ToWorkspace  VariableName=Liion_Charge1  SampleTime=1
  SoC Liion : ToWorkspace  VariableName=SoC_Liion1  SampleTime=1
  State of charge calulation : Subsystem
  Subsystem : Subsystem
  Initial Charge : Outport
  El consumption : Outport  Port=2
  El production : Outport  Port=3
  wires:
  El input/1 -> Ch eff/1, El consumption/1
  Subsystem/1("Initial charge ") -> Initial Charge/1
  El output/1 -> El production/1, 1/Dis eff/1
  State of charge calulation/1(State of Charege) -> SoC Liion/1
  Subsystem/2(New charge) -> State of charge calulation/1(Charge), Li-ion Charge/1
  Ch eff/1 -> Subsystem/1(El input)
  1/Dis eff/1 -> Subsystem/2(El output)

== system PLANET_v2/P2G/P2G ==
  El input : Inport
  Constant : Constant  Value=0
  Eff electrolyser : Gain  Gain=eff_electrolyser/100
  Eff methaniser : Gain  Gain=eff_methanizer/100
  Eff thermal : Gain  Gain=eff_thermal/100
  Max P2G electric input : Subsystem
  PCI : Gain  Gain=1/PCI
  Saturation Dynamic : simulink/Discontinuities/Saturation Dynamic  OutMin=0  OutMax=[]  OutDataTypeStr=Inherit: Same as second input  OutDataType=fixdt(1, 16)  OutScaling=2^-10  DoSatur=off
  Gas productioon : Outport
  El consumption : Outport  Port=2
  Heat production : Outport  Port=3
  wires:
  Max P2G electric input/1(Max P2G input) -> Saturation Dynamic/1
  Eff electrolyser/1 -> Eff methaniser/1  "H2 Power"
  Eff thermal/1 -> Heat production/1
  Eff methaniser/1 -> PCI/1  "CH4 Power"
  PCI/1 -> Gas productioon/1
  Saturation Dynamic/1 -> El consumption/1, Eff thermal/1, Eff electrolyser/1
  El input/1 -> Saturation Dynamic/2
  Constant/1 -> Saturation Dynamic/3

== system PLANET_v2/RES/Subsystem ==
  Wind : Inport
  PV : Inport  Port=2
  Hydro : Inport  Port=3
  RES1 : Outport
  RES2 : Outport  Port=2
  RES3 : Outport  Port=3
  wires:
  Wind/1 -> RES1/1
  PV/1 -> RES2/1
  Hydro/1 -> RES3/1

== system PLANET_v2/Subsystem/Environment ==
  Analogic control1 : Subsystem
  Analogic control2 : Subsystem
  Analogic control3 : Subsystem
  Bus Creator : BusCreator  Inputs=6
  Clock{2..4,6..7} (5 alike) : Clock
  Constant : Constant  Value=0
  Distric heat demand : Lookup_n-D  NumberOfTableDimensions=1  BreakpointsSpecification=Even spacing  BreakpointsForDimension1=tt  BreakpointsForDimension1FirstPoint=0  Table=dh_demand  InterpMethod=Flat  InternalRulePriority=Speed  RndMeth=Simplest  InputSameDT=on
  Hourly RES suplly profile1 : Lookup_n-D  NumberOfTableDimensions=1  BreakpointsSpecification=Even spacing  BreakpointsForDimension1=tt  BreakpointsForDimension1FirstPoint=0  Table=WindPower  InterpMethod=Flat  InternalRulePriority=Speed  RndMeth=Simplest  InputSameDT=on
  "Hourly RES suplly profile2 " : Lookup_n-D  NumberOfTableDimensions=1  BreakpointsSpecification=Even spacing  BreakpointsForDimension1=tt  BreakpointsForDimension1FirstPoint=0  Table=PVPower  InterpMethod=Flat  InternalRulePriority=Speed  RndMeth=Simplest  InputSameDT=on
  Hourly electric demand profile1 : Lookup_n-D  NumberOfTableDimensions=1  BreakpointsSpecification=Even spacing  BreakpointsForDimension1=tt  BreakpointsForDimension1FirstPoint=0  Table=h_elD  InterpMethod=Flat  InternalRulePriority=Speed  RndMeth=Simplest  InputSameDT=on
  Local heat demand : Lookup_n-D  NumberOfTableDimensions=1  BreakpointsSpecification=Even spacing  BreakpointsForDimension1=tt  BreakpointsForDimension1FirstPoint=0  Table=lhd_demand  InterpMethod=Flat  InternalRulePriority=Speed  RndMeth=Simplest  InputSameDT=on
  Environmental conditions : Outport
  wires:
  Clock2/1 -> Hourly RES suplly profile1/1
  Clock3/1 -> Hourly electric demand profile1/1
  Clock4/1 -> "Hourly RES suplly profile2 "/1
  Hourly electric demand profile1/1 -> Bus Creator/1  "El dem"
  Bus Creator/1 -> Environmental conditions/1
  "Hourly RES suplly profile2 "/1 -> Analogic control2/1(Value)
  Hourly RES suplly profile1/1 -> Analogic control1/1(Value)
  Analogic control2/1(Modifed value) -> Bus Creator/5  "PV"
  Analogic control1/1(Modifed value) -> Bus Creator/4  "Wind"
  Clock6/1 -> Distric heat demand/1
  Clock7/1 -> Local heat demand/1
  Distric heat demand/1 -> Bus Creator/2  "DH standar profile"
  Local heat demand/1 -> Bus Creator/3  "LH standard profile"
  Analogic control3/1(Modifed value) -> Bus Creator/6  "Hydro"
  Constant/1 -> Analogic control3/1(Value)

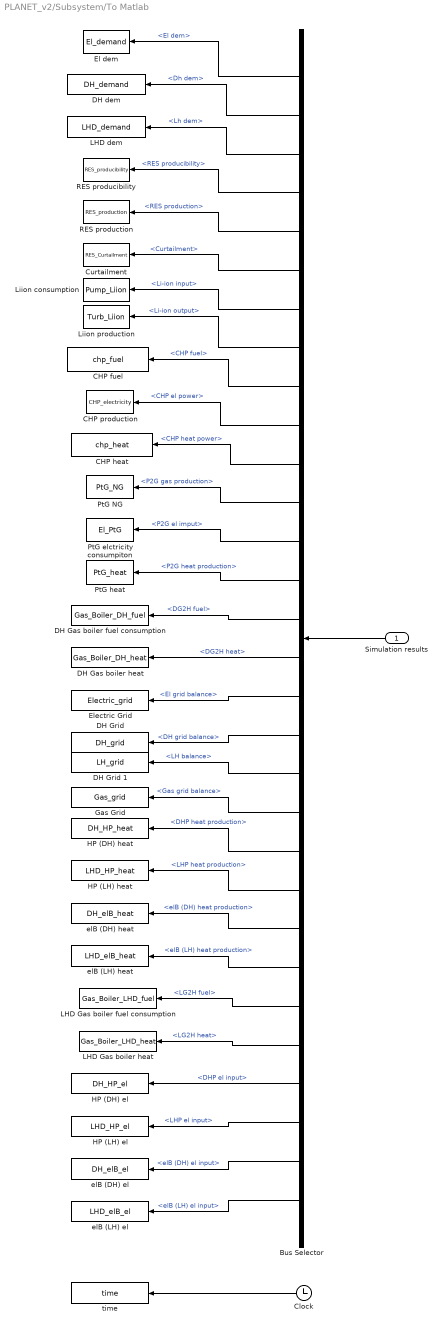
== system PLANET_v2/Subsystem/To Matlab ==
  Simulation results : Inport
  Bus Selector : BusSelector  OutputSignals=Energy demand.El dem,Energy demand.Thermal demand.Dh dem,Energy demand.Thermal demand.Lh dem,RES.RES producibility,RES.RES production,RES.Curtailment,Li-ion signals.Li-ion input,Li-ion signals.Li-ion output,CHP signals.CHP fuel,CHP signals.CHP el power,CHP signals.CHP heat power,P2G signals.P2G gas production,P2G signals.P2G el imput,P2G signals.P2G heat production,G2H (DH) data.DG2H fuel,G2H (DH) data.DG2H heat,Grid balance.El grid balance,Grid balance.DH grid balance,Grid balance.LH balance,Grid balance.Gas grid balance,HP (DH) data.DHP heat production,HP (LH) data.LHP heat production,elB (DH) data.elB (DH) heat production,elB (LH) data.elB (LH) heat production,G2H (LH) data.LG2H fuel,G2H (LH) data.LG2H heat,HP (DH) data.DHP el input,HP (LH) data.LHP el input,elB (DH) data.elB (DH) el input,elB (LH) data.elB (LH) el input
  CHP fuel : ToWorkspace  VariableName=chp_fuel  SampleTime=1
  CHP heat : ToWorkspace  VariableName=chp_heat  SampleTime=1
  CHP production : ToWorkspace  VariableName=CHP_electricity  SampleTime=1
  Clock : Clock
  Curtailment : ToWorkspace  VariableName=RES_Curtailment  SampleTime=1
  DH Gas boiler fuel consumption : ToWorkspace  VariableName=Gas_Boiler_DH_fuel  SampleTime=1
  DH Gas boiler heat : ToWorkspace  VariableName=Gas_Boiler_DH_heat  SampleTime=1
  "DH Grid " : ToWorkspace  VariableName=DH_grid  SampleTime=1
  DH Grid 1 : ToWorkspace  VariableName=LH_grid  SampleTime=1
  DH dem : ToWorkspace  VariableName=DH_demand  SampleTime=1
  El dem : ToWorkspace  VariableName=El_demand  SampleTime=1
  Electric Grid : ToWorkspace  VariableName=Electric_grid  SampleTime=1
  "Gas Grid " : ToWorkspace  VariableName=Gas_grid  SampleTime=1
  HP (DH) el : ToWorkspace  VariableName=DH_HP_el  SampleTime=1
  HP (DH) heat : ToWorkspace  VariableName=DH_HP_heat  SampleTime=1
  HP (LH) el : ToWorkspace  VariableName=LHD_HP_el  SampleTime=1
  HP (LH) heat : ToWorkspace  VariableName=LHD_HP_heat  SampleTime=1
  LHD Gas boiler fuel consumption : ToWorkspace  VariableName=Gas_Boiler_LHD_fuel  SampleTime=1
  LHD Gas boiler heat : ToWorkspace  VariableName=Gas_Boiler_LHD_heat  SampleTime=1
  LHD dem : ToWorkspace  VariableName=LHD_demand  SampleTime=1
  Liion consumption : ToWorkspace  VariableName=Pump_Liion  SampleTime=1
  Liion production : ToWorkspace  VariableName=Turb_Liion  SampleTime=1
  PtG NG : ToWorkspace  VariableName=PtG_NG  SampleTime=1
  PtG elctricity consumpiton : ToWorkspace  VariableName=El_PtG  SampleTime=1
  PtG heat : ToWorkspace  VariableName=PtG_heat  SampleTime=1
  RES producibility : ToWorkspace  VariableName=RES_producibility  SampleTime=1
  RES production : ToWorkspace  VariableName=RES_production  SampleTime=1
  elB (DH) el : ToWorkspace  VariableName=DH_elB_el  SampleTime=1
  elB (DH) heat : ToWorkspace  VariableName=DH_elB_heat  SampleTime=1
  elB (LH) el : ToWorkspace  VariableName=LHD_elB_el  SampleTime=1
  elB (LH) heat : ToWorkspace  VariableName=LHD_elB_heat  SampleTime=1
  time : ToWorkspace  VariableName=time  SampleTime=1
  wires:
  Bus Selector/5 -> RES production/1  "<RES production>"
  Bus Selector/20 -> "Gas Grid "/1  "<Gas grid balance>"
  Bus Selector/17 -> Electric Grid/1  "<El grid balance>"
  Bus Selector/18 -> "DH Grid "/1  "<DH grid balance>"
  Bus Selector/8 -> Liion production/1  "<Li-ion output>"
  Bus Selector/7 -> Liion consumption/1  "<Li-ion input>"
  Bus Selector/9 -> CHP fuel/1  "<CHP fuel>"
  Bus Selector/14 -> PtG heat/1  "<P2G heat production>"
  Bus Selector/13 -> PtG elctricity consumpiton/1  "<P2G el imput>"
  Bus Selector/11 -> CHP heat/1  "<CHP heat power>"
  Bus Selector/10 -> CHP production/1  "<CHP el power>"
  Bus Selector/12 -> PtG NG/1  "<P2G gas production>"
  Bus Selector/15 -> DH Gas boiler fuel consumption/1  "<DG2H fuel>"
  Bus Selector/16 -> DH Gas boiler heat/1  "<DG2H heat>"
  Bus Selector/1 -> El dem/1  "<El dem>"
  Bus Selector/2 -> DH dem/1  "<Dh dem>"
  Bus Selector/4 -> RES producibility/1  "<RES producibility>"
  Simulation results/1 -> Bus Selector/1
  Bus Selector/24 -> elB (LH) heat/1  "<elB (LH) heat production>"
  Bus Selector/21 -> HP (DH) heat/1  "<DHP heat production>"
  Bus Selector/22 -> HP (LH) heat/1  "<LHP heat production>"
  Bus Selector/23 -> elB (DH) heat/1  "<elB (DH) heat production>"
  Bus Selector/25 -> LHD Gas boiler fuel consumption/1  "<LG2H fuel>"
  Bus Selector/26 -> LHD Gas boiler heat/1  "<LG2H heat>"
  Bus Selector/29 -> elB (DH) el/1  "<elB (DH) el input>"
  Bus Selector/28 -> HP (LH) el/1  "<LHP el input>"
  Bus Selector/27 -> HP (DH) el/1  "<DHP el input>"
  Bus Selector/30 -> elB (LH) el/1  "<elB (LH) el input>"
  Bus Selector/6 -> Curtailment/1  "<Curtailment>"
  Bus Selector/3 -> LHD dem/1  "<Lh dem>"
  Bus Selector/19 -> DH Grid 1/1  "<LH balance>"
  Clock/1 -> time/1

== system PLANET_v2/Subsystem2/Distric heating grid ==
  Demand consumption : Inport
  CHP production : Inport  Port=2
  P2G production : Inport  Port=3
  Gas boiler (DH) : Inport  Port=4
  HP (DH) : Inport  Port=5
  El B (DH) : Inport  Port=6
  Bus Selector1 : BusSelector  OutputSignals=CHP heat power
  Bus Selector2 : BusSelector  OutputSignals=P2G heat production
  Bus Selector3 : BusSelector  OutputSignals=Thermal demand.Dh dem
  Bus Selector4 : BusSelector  OutputSignals=elB (DH) heat production
  Bus Selector5 : BusSelector  OutputSignals=DG2H heat
  Bus Selector6 : BusSelector  OutputSignals=DHP heat production
  Sum : Sum  Inputs=+++++|-
  Distric heating balance : Outport
  wires:
  CHP production/1 -> Bus Selector1/1
  P2G production/1 -> Bus Selector2/1
  Gas boiler (DH)/1 -> Bus Selector5/1
  Demand consumption/1 -> Bus Selector3/1
  Sum/1 -> Distric heating balance/1
  HP (DH)/1 -> Bus Selector6/1
  Bus Selector6/1 -> Sum/4  "<DHP heat production>"
  Bus Selector5/1 -> Sum/3  "<DG2H heat>"
  Bus Selector1/1 -> Sum/1  "<CHP heat power>"
  Bus Selector2/1 -> Sum/2  "<P2G heat production>"
  Bus Selector3/1 -> Sum/6  "<Dh dem>"
  El B (DH)/1 -> Bus Selector4/1
  Bus Selector4/1 -> Sum/5  "<elB (DH) heat production>"

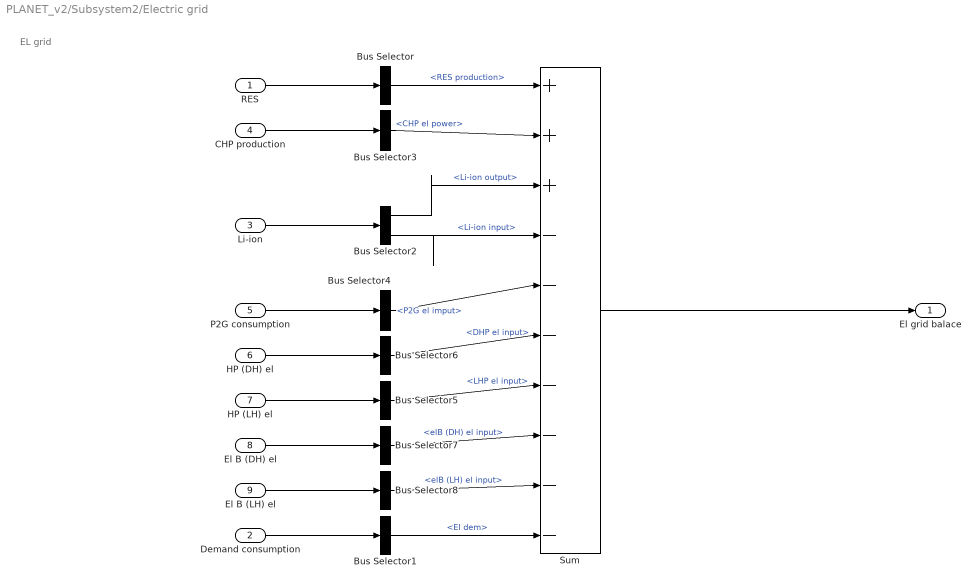
== system PLANET_v2/Subsystem2/Electric grid ==
  note: EL grid
  RES : Inport
  Demand consumption : Inport  Port=2
  Li-ion : Inport  Port=3
  CHP production : Inport  Port=4
  P2G consumption : Inport  Port=5
  HP (DH) el : Inport  Port=6
  HP (LH) el : Inport  Port=7
  El B (DH) el : Inport  Port=8
  El B (LH) el : Inport  Port=9
  Bus Selector : BusSelector  OutputSignals=RES production
  Bus Selector1 : BusSelector  OutputSignals=El dem
  Bus Selector2 : BusSelector  OutputSignals=Li-ion output,Li-ion input
  Bus Selector3 : BusSelector  OutputSignals=CHP el power
  Bus Selector4 : BusSelector  OutputSignals=P2G el imput
  Bus Selector5 : BusSelector  OutputSignals=LHP el input
  Bus Selector6 : BusSelector  OutputSignals=DHP el input
  Bus Selector7 : BusSelector  OutputSignals=elB (DH) el input
  Bus Selector8 : BusSelector  OutputSignals=elB (LH) el input
  Sum : Sum  Inputs=+++|-------
  El grid balace : Outport
  wires:
  RES/1 -> Bus Selector/1
  Li-ion/1 -> Bus Selector2/1
  CHP production/1 -> Bus Selector3/1
  P2G consumption/1 -> Bus Selector4/1
  Demand consumption/1 -> Bus Selector1/1
  Sum/1 -> El grid balace/1
  HP (DH) el/1 -> Bus Selector6/1
  Bus Selector/1 -> Sum/1  "<RES production>"
  Bus Selector1/1 -> Sum/10  "<El dem>"
  Bus Selector2/2 -> Sum/4  "<Li-ion input>"
  Bus Selector2/1 -> Sum/3  "<Li-ion output>"
  Bus Selector3/1 -> Sum/2  "<CHP el power>"
  Bus Selector4/1 -> Sum/5  "<P2G el imput>"
  Bus Selector6/1 -> Sum/6  "<DHP el input>"
  Bus Selector5/1 -> Sum/7  "<LHP el input>"
  HP (LH) el/1 -> Bus Selector5/1
  Bus Selector7/1 -> Sum/8  "<elB (DH) el input>"
  El B (DH) el/1 -> Bus Selector7/1
  Bus Selector8/1 -> Sum/9  "<elB (LH) el input>"
  El B (LH) el/1 -> Bus Selector8/1

== system PLANET_v2/Subsystem2/Gas grid ==
  CHP consumption : Inport
  P2G production : Inport  Port=2
  Gas boiler (DH) : Inport  Port=3
  Gas boiler (LH) : Inport  Port=4
  Bus Selector1 : BusSelector  OutputSignals=P2G gas production
  Bus Selector2 : BusSelector  OutputSignals=CHP fuel
  Bus Selector3 : BusSelector  OutputSignals=LG2H fuel
  Bus Selector5 : BusSelector  OutputSignals=DG2H fuel
  Sum : Sum  Inputs=+|---
  Gas grid balance : Outport
  wires:
  CHP consumption/1 -> Bus Selector2/1
  P2G production/1 -> Bus Selector1/1
  Gas boiler (DH)/1 -> Bus Selector5/1
  Sum/1 -> Gas grid balance/1
  Bus Selector5/1 -> Sum/2  "<DG2H fuel>"
  Bus Selector1/1 -> Sum/1  "<P2G gas production>"
  Bus Selector2/1 -> Sum/4  "<CHP fuel>"
  Gas boiler (LH)/1 -> Bus Selector3/1
  Bus Selector3/1 -> Sum/3  "<LG2H fuel>"

== system PLANET_v2/Subsystem2/Local heat ==
  LH dem : Inport
  Gas boiler (LH) : Inport  Port=2
  HP (LH) : Inport  Port=3
  El B (LH) : Inport  Port=4
  Bus Selector1 : BusSelector  OutputSignals=LHP heat production
  Bus Selector2 : BusSelector  OutputSignals=Thermal demand.Lh dem
  Bus Selector3 : BusSelector  OutputSignals=LG2H heat
  Bus Selector5 : BusSelector  OutputSignals=elB (LH) heat production
  Scope : Scope
  Sum : Sum  Inputs=+++|-
  LH balance : Outport
  wires:
  LH dem/1 -> Bus Selector2/1
  HP (LH)/1 -> Bus Selector1/1
  El B (LH)/1 -> Bus Selector5/1
  Sum/1 -> LH balance/1
  Bus Selector5/1 -> Scope/1, Sum/3  "<elB (LH) heat production>"
  Bus Selector1/1 -> Sum/2  "<LHP heat production>"
  Bus Selector2/1 -> Sum/4  "<Lh dem>"
  Gas boiler (LH)/1 -> Bus Selector3/1
  Bus Selector3/1 -> Sum/1  "<LG2H heat>"

== system PLANET_v2/CHP/CHP /CHP ==
  Fuel mass flow rate : Inport
  Divide1 : Product  Inputs=***
  Divide2 : Product  Inputs=***
  Electric efficiency : Constant  Value=eff_el/100
  Internal comsumption : Constant  Value=Paus
  PCI MJ/kg1 : Constant  Value=PCI
  PCI MJ/kg2 : Constant  Value=PCI
  Sum1 : Sum  Inputs=|+-|
  Thermal efficiency : Constant  Value=eff_th/100
  Electric power : Outport
  Thermal power : Outport  Port=2
  wires:
  PCI MJ/kg2/1 -> Divide1/2
  Fuel mass flow rate/1 -> Divide2/1, Divide1/1
  Divide2/1 -> Sum1/1
  Thermal efficiency/1 -> Divide1/3
  Sum1/1 -> Electric power/1
  Electric efficiency/1 -> Divide2/3
  PCI MJ/kg1/1 -> Divide2/2
  Internal comsumption/1 -> Sum1/2
  Divide1/1 -> Thermal power/1

== system PLANET_v2/Control /Li-ion control/Available Energy MWh ==
  In1 : Inport
  Capacity [MWh] : Constant  Value=Capacity
  Product1 : Product
  Steate of Charge MIN : Constant  Value=SoC_MIN/100
  Sum : Sum  Inputs=+|-
  Charge available : Outport
  wires:
  Sum/1 -> Charge available/1
  Steate of Charge MIN/1 -> Product1/2
  Capacity [MWh]/1 -> Product1/1
  In1/1 -> Sum/1
  Product1/1 -> Sum/2

== system PLANET_v2/Control /Li-ion control/Energy to Power ==
  Energy : Inport
  Energy to Power : Gain  Gain=1/dt
  Power : Outport
  wires:
  Energy/1 -> Energy to Power/1
  Energy to Power/1 -> Power/1

== system PLANET_v2/Control /Li-ion control/If Action Subsystem3 ==
  Action Port : ActionPort  ActionType=then
  Constant : Constant  Value=0
  From battery : Outport
  "Bypassed demand " : Outport  Port=2
  wires:
  Constant/1 -> "Bypassed demand "/1, From battery/1

== system PLANET_v2/Control /Li-ion control/If Action Subsystem5 ==
  Demand : Inport
  Action Port : ActionPort  ActionType=elseif
  Constant : Constant  Value=0
  From battery : Outport
  Bypassed demand : Outport  Port=2
  wires:
  Demand/1 -> From battery/1
  Constant/1 -> Bypassed demand/1

== system PLANET_v2/Control /Li-ion control/If Action Subsystem6 ==
  Max discharge : Inport
  Demand : Inport  Port=2
  Action Port : ActionPort  ActionType=elseif
  Sum : Sum  Inputs=-+|
  From battery : Outport
  Bypassed demand : Outport  Port=2
  wires:
  Max discharge/1 -> Sum/1, From battery/1
  Demand/1 -> Sum/2
  Sum/1 -> Bypassed demand/1

== system PLANET_v2/Control /Li-ion control/If Action Subsystem7 ==
  Available battery : Inport
  Demnad : Inport  Port=2
  Action Port : ActionPort  ActionType=else
  Sum : Sum  Inputs=-+|
  From battery : Outport
  Bypassed demand : Outport  Port=2
  wires:
  Available battery/1 -> Sum/1, From battery/1
  Demnad/1 -> Sum/2
  Sum/1 -> Bypassed demand/1
